simulink model "sistema_stabilizzato"  (R2025b)
settings: Solver=ode45  StartTime=0.0  StopTime=10  RelTol=1e-3
libraries: cstblocks x1
settings Model: Creator=USER  LastModifiedBy=francesco
settings SolverCC: AlgebraicLoopSolver=TrustRegion
settings DebuggingCC: UnconnectedInputMsg=warning  UnconnectedOutputMsg=warning  UnconnectedLineMsg=warning
settings ModelReferenceCC: EnableRefExpFcnMdlSchedulingChecks=on
settings RTWCC: GPUComputeCapability=3.5  DLArmComputeVersion=19.05

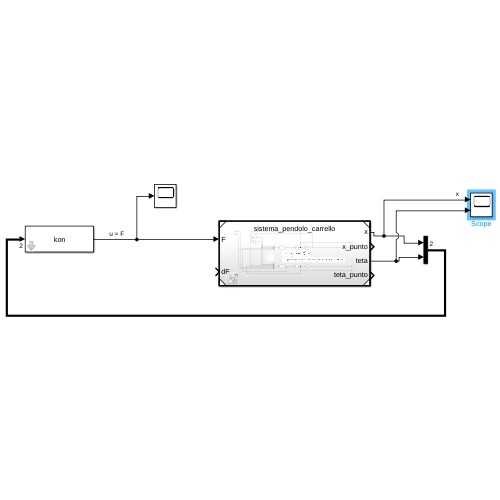
[thumbnail: Simulink's stored preview of the top-level diagram]
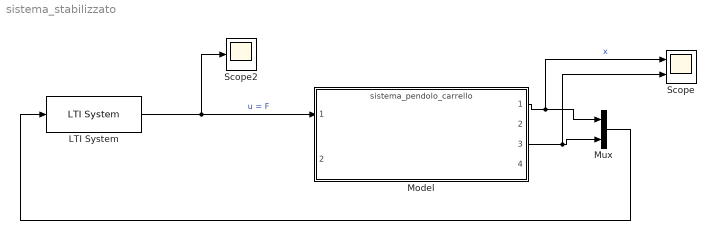
== system sistema_stabilizzato ==
  LTI System : cstblocks/LTI System  sys=kon  IC=[]  PadeOrder=0
  Model : ModelReference  ModelNameDialog=sistema_pendolo_carrello.slx  SimulationMode=Normal  ModelReferenceVersion=9.24
  Mux : Mux  Inputs=2
  Scope : Scope  NumInputPorts=2
      settings: ActiveDisplayYMinimum=-0.049032264504971432  ActiveDisplayYMaximum=0.11655922772141601
  Scope2 : Scope
      settings: ActiveDisplayYMinimum=-2.3539281040749657E+10  ActiveDisplayYMaximum=2.1185352929157202E+11  DataLoggingVariableName=ScopeData2
  wires:
  LTI System/1 -> Scope2/1, Model/1  "u = F"
  Model/1 -> Mux/1, Scope/1  "x"
  Mux/1 -> LTI System/1
  Model/3 -> Mux/2, Scope/2
